simulink model "Example_heat"  (R2015b)
settings: Solver=ode45  SolverMode=SingleTasking  StartTime=0.0  StopTime=48  FixedStep=1  RelTol=1e-3  AbsTol=1e-6
model workspace (MATLAB code in the model file):
  | % load initial conditions and physical properties from file
  | 
  | sldemo_househeat_data
values from neighbouring files (symbols this model uses):
  a = str2double (get(handles.tem, 'string'))    [temperature.m]
  b = str2double (get(handles.avetem, 'string'))    [temperature.m]
undefined symbols (not defined in the file or in its folder): c, M, Mdot, Req, THeater, TinIC
Description:
  | Thermal Model of a House
  | 
  | This demo illustrates how you can use Simulink(R) to create the thermal model of
  | a house. This system models the outdoor environment, the thermal
  | characteristics of the house, and the house heating system.
  | 
  | The sldemo_househeat_data.m file initializes data in the model workspace.
  | To make changes, you can edit the model workspace directly or edit the MATLAB(R) file
  | and re-load the model workspace.
  | 
  | To view the model workspace, select View > Model Explorer
  | from the Simulink editor.
  | 
  | Note: Time is given in units of hours
settings Model: ExtModeTrigMode=oneshot  ExtModeArmWhenConnect=off  ExtModeAutoUpdateStatusClock=off  Creator=The MathWorks, Inc.  LastModifiedBy=mctra
settings DataIOCC: ExternalInput=[]  InitialState=[]  LimitDataPoints=off  SaveFormat=Array  SaveOutput=off  SaveTime=off  SignalLoggingName=sldemo_househeat_output
settings OptimizationCC: BlockReduction=off  BooleanDataType=off  ExpressionDepthLimit=2147483647  InitFltsAndDblsToZero=on  BufferReusableBoundary=off
settings DebuggingCC: SaveWithParameterizedLinksMsg=none  UnderspecifiedInitializationDetection=Classic  MergeDetectMultiDrivingBlocksExec=none  SignalResolutionControl=TryResolveAllWithWarning  MultiTaskDSMMsg=warning  MultiTaskCondExecSysMsg=none  IntegerOverflowMsg=none  FcnCallInpInsideContextMsg=UseLocalSettings  BusObjectLabelMismatch=none  StateNameClashWarn=warning  IntegerSaturationMsg=none
settings HardwareCC: ProdBitPerPointer=32  ProdLargestAtomicFloat=None  ProdIntDivRoundTo=Undefined  ProdEndianess=Unspecified  ProdWordSize=32  ProdHWDeviceType=32-bit Generic  TargetUnknown=on
settings GRTTargetCC: TargetFcnLib=ansi_tfl_tmw.mat  GeneratePreprocessorConditionals=Disable all  CombineOutputUpdateFcns=off  GRTInterface=on
settings ConfigComp: CovModelRefEnable=Off

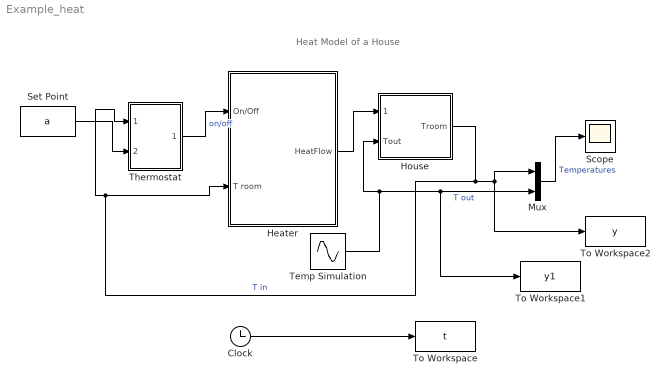
== system Example_heat ==
  note: Heat Model of a House
  Clock : Clock
  Heater : Subsystem
      mask Display: image('heater-128.jpg')
  House : Subsystem
      mask Display: image('icons_ps_house-flat.jpg')
  Mux : Mux  Inputs=2
  Scope : Scope
  Set Point : Constant  Value=a
  Temp Simulation : Sin  Amplitude=10  Bias=b  Frequency=2*pi/24  SampleTime=0
  Thermostat : Subsystem
      mask Display: image('switch-button-54069.jpg')
  To Workspace : ToWorkspace  VariableName=t  SampleTime=-1
  To Workspace1 : ToWorkspace  VariableName=y1  SampleTime=-1
  To Workspace2 : ToWorkspace  VariableName=y  SampleTime=-1
  wires:
  Thermostat/1(switch) -> Heater/1(On/Off)  "on/off"
  House/1(Troom) -> Thermostat/1(room temperature), Heater/2(T room), To Workspace2/1, Mux/1  "T in"
  Heater/1(HeatFlow) -> House/1(Heater dQ gain / dt)
  Set Point/1 -> Thermostat/2(set room temperature)
  Mux/1 -> Scope/1  "Temperatures"
  Clock/1 -> To Workspace/1
  Temp Simulation/1 -> House/2(Tout), To Workspace1/1, Mux/2  "T out"

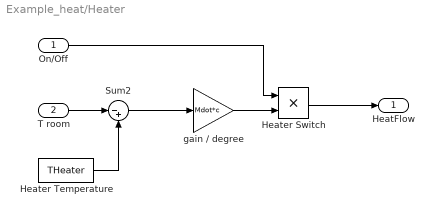
== system Example_heat/Heater ==
  On/Off : Inport
  T room : Inport  Port=2
  Heater Switch : Product  RndMeth=Zero
  Heater Temperature : Constant  Value=THeater
  Sum2 : Sum  Inputs=|-+
  gain / degree : Gain  Gain=Mdot*c
  HeatFlow : Outport
  wires:
  Heater Temperature/1 -> Sum2/2
  T room/1 -> Sum2/1
  Sum2/1 -> gain / degree/1
  On/Off/1 -> Heater Switch/1
  gain / degree/1 -> Heater Switch/2
  Heater Switch/1 -> HeatFlow/1

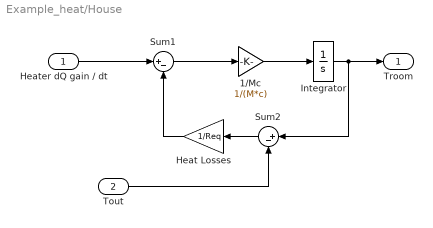
== system Example_heat/House ==
  Heater dQ gain / dt : Inport
  Tout : Inport  Port=2
  1/Mc : Gain  Gain=1/(M*c)  SaturateOnIntegerOverflow=on  OutDataTypeStr=Inherit: Same as input  ParamDataTypeStr=Inherit: Same as input
  Heat Losses : Gain  Gain=1/Req  SaturateOnIntegerOverflow=on  OutDataTypeStr=Inherit: Same as input  ParamDataTypeStr=Inherit: Same as input
  Integrator : Integrator  InitialCondition=TinIC
  Sum1 : Sum  Inputs=|+-  SaturateOnIntegerOverflow=on  InputSameDT=on  OutDataTypeStr=Inherit: Same as first input
  Sum2 : Sum  Inputs=|+-  SaturateOnIntegerOverflow=on  InputSameDT=on  OutDataTypeStr=Inherit: Same as first input
  Troom : Outport  InitialOutput=0
  wires:
  Tout/1 -> Sum2/2
  Heater dQ gain / dt/1 -> Sum1/1
  Sum1/1 -> 1/Mc/1
  Sum2/1 -> Heat Losses/1
  Heat Losses/1 -> Sum1/2
  1/Mc/1 -> Integrator/1
  Integrator/1 -> Sum2/1, Troom/1

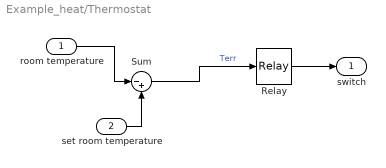
== system Example_heat/Thermostat ==
  room temperature : Inport
  set room temperature : Inport  Port=2
  Relay : Relay  OnSwitchValue=2  OffSwitchValue=-2
  Sum : Sum  Inputs=|-+
  switch : Outport  InitialOutput=0
  wires:
  Relay/1 -> switch/1
  Sum/1 -> Relay/1  "Terr"
  room temperature/1 -> Sum/1
  set room temperature/1 -> Sum/2
